simulink model "TVModel_Simulation"  (R2022a)
settings: Solver=FixedStepDiscrete  StartTime=0.0  StopTime=200  FixedStep=0.02  MaxStep=0.01  RelTol=1e-3
undefined symbols (not defined in the file or in its folder): TV
libraries: simulink x5, simulink_extras x3, dspstat3 x2, sharedTrackingLibrary x1, slpidlib x1, eeGeneralControl x1
(part 2 of 4)

== system TVModel_Simulation/Subsystem/Subsystem1/Slip Control/Slip Ratios/FR SR ==
  In Bus Element : Inport  PortName=dynamics_data  Element=omega_wheels
  In Bus Element4 : Inport  PortName=dynamics_data  Element=vx
  In Bus Element2 : Inport  PortName=dynamics_data  Element=vx
  In Bus Element1 : Inport  PortName=dynamics_data  Element=vy
  In Bus Element6 : Inport  Port=2  PortName=front_wheels_steering  Element=different_axis
  Constant : Constant  Value=0
  Cos1 : Trigonometry  Operator=cos
  Cos2 : Trigonometry
  Divide4 : Product  Inputs=*/
  Divide5 : Product  Inputs=**
  Divide6 : Product  Inputs=**
  Gain3 : Gain  Gain=TV.CAR.rs
  Selector : Selector  InputPortWidth=4  IndexOptions=Index vector (dialog)  Indices=[2]  OutputSizes=1
  Selector1 : Selector  InputPortWidth=2  IndexOptions=Index vector (dialog)  Indices=[2]  OutputSizes=1
  Subtract3 : Sum  Inputs=+-
  Sum : Sum
  Switch : Switch  Criteria=u2 > Threshold  Threshold=0.5  SaturateOnIntegerOverflow=off  InputSameDT=off
  FR : Outport
  wires:
  Constant/1 -> Switch/3
  Divide4/1 -> Switch/1  "FL"
  In Bus Element1/1 -> Divide6/2
  In Bus Element2/1 -> Divide5/1
  Divide6/1 -> Sum/2
  Gain3/1 -> Subtract3/1
  Divide5/1 -> Sum/1
  Cos1/1 -> Divide5/2
  Sum/1 -> Subtract3/2, Divide4/2
  Cos2/1 -> Divide6/1
  Subtract3/1 -> Divide4/1
  Switch/1 -> FR/1
  In Bus Element/1 -> Selector/1  "fr"
  Selector/1 -> Gain3/1
  In Bus Element4/1 -> Switch/2
  Selector1/1 -> Cos2/1, Cos1/1
  In Bus Element6/1 -> Selector1/1

== system TVModel_Simulation/Subsystem/Subsystem1/Slip Control/Slip Ratios/RL RR  ==
  In Bus Element : Inport  PortName=dynamics_data  Element=omega_wheels
  In Bus Element1 : Inport  PortName=dynamics_data  Element=vx
  Constant : Constant  Value=0
  Divide : Product  Inputs=*/
  Gain : Gain  Gain=TV.CAR.rs
  Selector : Selector  InputPortWidth=4  IndexOptions=Index vector (dialog)  Indices=[4]  OutputSizes=1
  Subtract : Sum  Inputs=+-
  Switch : Switch  Criteria=u2 > Threshold  Threshold=0.5  SaturateOnIntegerOverflow=off  InputSameDT=off
  RR : Outport
  wires:
  Constant/1 -> Switch/3
  Divide/1 -> Switch/1  "RL"
  Switch/1 -> RR/1  "RR"
  Gain/1 -> Subtract/1
  Subtract/1 -> Divide/1
  In Bus Element1/1 -> Switch/2, Divide/2, Subtract/2
  In Bus Element/1 -> Selector/1  "rr"
  Selector/1 -> Gain/1

== system TVModel_Simulation/Subsystem/Subsystem1/Slip Control/Slip Ratios/RL SR ==
  In Bus Element : Inport  PortName=dynamics_data  Element=omega_wheels
  In Bus Element1 : Inport  PortName=dynamics_data  Element=vx
  Constant : Constant  Value=0
  Divide : Product  Inputs=*/
  Gain : Gain  Gain=TV.CAR.rs
  Selector : Selector  InputPortWidth=4  IndexOptions=Index vector (dialog)  Indices=[3]  OutputSizes=1
  Subtract : Sum  Inputs=+-
  Switch : Switch  Criteria=u2 > Threshold  Threshold=0.5  SaturateOnIntegerOverflow=off  InputSameDT=off
  RL : Outport
  wires:
  In Bus Element1/1 -> Subtract/2, Divide/2, Switch/2
  Subtract/1 -> Divide/1
  Gain/1 -> Subtract/1
  Switch/1 -> RL/1  "RL"
  Divide/1 -> Switch/1  "RL"
  Constant/1 -> Switch/3
  In Bus Element/1 -> Selector/1  "rl"
  Selector/1 -> Gain/1

== system TVModel_Simulation/Subsystem/Subsystem1/Torque Distribution/MPC/     Output vector reference ==
  YRD : Inport
  In Bus Element1 : Inport  Port=2  PortName=dynamics_data  Element=vy
  In Bus Element : Inport  Port=2  PortName=dynamics_data  Element=vx
  In Bus Element3 : Inport  Port=2  PortName=dynamics_data  Element=vx
  In Bus Element2 : Inport  Port=3  PortName=driver_inputs  Element=throttle
  Bus Creator : BusCreator  Inputs=11
  Bus y_ref : Subsystem
  MATLAB Function : MATLAB Function  TreatAsAtomicUnit=on
  MATLAB Function1 : MATLAB Function  TreatAsAtomicUnit=on
  T_FL_ref : Constant  Value=0
  T_FR_ref : Constant  Value=0
  T_RL_ref : Constant  Value=0
  T_RR_ref : Constant  Value=0
  YRD1 : InportShadow
  dT_FL_ref : Constant  Value=0
  dT_FR_ref : Constant  Value=0
  dT_RL_ref : Constant  Value=0
  dT_RR_ref : Constant  Value=0
  y_ref_0 : Outport
  y_ref : Outport  Port=2
  Out Bus Element5 : Outport  Port=3  PortName=TV_Info  Element=vx_ref
  Out Bus Element1 : Outport  Port=3  PortName=TV_Info  Element=vy_ref
  wires:
  dT_RR_ref/1 -> Bus Creator/11
  dT_RL_ref/1 -> Bus Creator/10
  dT_FR_ref/1 -> Bus Creator/9
  dT_FL_ref/1 -> Bus Creator/8
  In Bus Element2/1 -> MATLAB Function1/3(acc)
  In Bus Element1/1 -> MATLAB Function1/2(vy)
  In Bus Element/1 -> MATLAB Function1/1(vx)
  MATLAB Function1/1(vx_ref) -> Bus Creator/1, Out Bus Element5/1  "vx_ref"
  MATLAB Function/1(vy_ref) -> Bus Creator/2, Out Bus Element1/1  "vy_ref"
  T_FL_ref/1 -> Bus Creator/4
  T_FR_ref/1 -> Bus Creator/5
  T_RL_ref/1 -> Bus Creator/6
  T_RR_ref/1 -> Bus Creator/7
  Bus Creator/1 -> Bus y_ref/1(u), y_ref_0/1
  Bus y_ref/1(y) -> y_ref/1
  In Bus Element3/1 -> MATLAB Function/1(vx)
  YRD/1 -> MATLAB Function/2(YRD)  "r_ref"
  YRD1/1 -> Bus Creator/3  "r_ref"

== system TVModel_Simulation/Subsystem/Subsystem1/Torque Distribution/MPC/ Parameter Bus  ==
  note: Nominal LMU = 0.93
  In Bus Element1 : Inport  PortName=slip_ratio  Element=fl
  In Bus Element2 : Inport  PortName=slip_ratio  Element=fr
  In Bus Element3 : Inport  PortName=slip_ratio  Element=rl
  In Bus Element4 : Inport  PortName=slip_ratio  Element=rr
  In Bus Element5 : Inport  Port=2  PortName=dynamics_data  Element=ax
  In Bus Element6 : Inport  Port=2  PortName=dynamics_data  Element=ay
  In Bus Element12 : Inport  Port=2  PortName=dynamics_data  Element=brake_torque
  In Bus Element11 : Inport  Port=3  PortName=front_wheel_angles  Element=single_axis
  Bus p : Subsystem
  Demux : Demux
  Inertia Scaling : Constant
  LMUy : Constant  Value=0.93
  Mux : Mux  Inputs=TV.MPC.np
  Signal Specification{4..7} (4 alike) : SignalSpecification  Dimensions=1
  p : Outport
  wires:
  Inertia Scaling/1 -> Mux/13
  In Bus Element11/1 -> Mux/1
  LMUy/1 -> Mux/12
  Bus p/1(Out) -> p/1
  Demux/1 -> Signal Specification4/1
  Demux/2 -> Signal Specification5/1
  Demux/3 -> Signal Specification6/1
  Demux/4 -> Signal Specification7/1
  Signal Specification4/1 -> Mux/6
  Signal Specification5/1 -> Mux/7
  Signal Specification6/1 -> Mux/8
  Signal Specification7/1 -> Mux/9
  Mux/1 -> Bus p/1(In)
  In Bus Element1/1 -> Mux/2
  In Bus Element4/1 -> Mux/5
  In Bus Element3/1 -> Mux/4
  In Bus Element2/1 -> Mux/3
  In Bus Element6/1 -> Mux/10
  In Bus Element5/1 -> Mux/11
  In Bus Element12/1 -> Demux/1

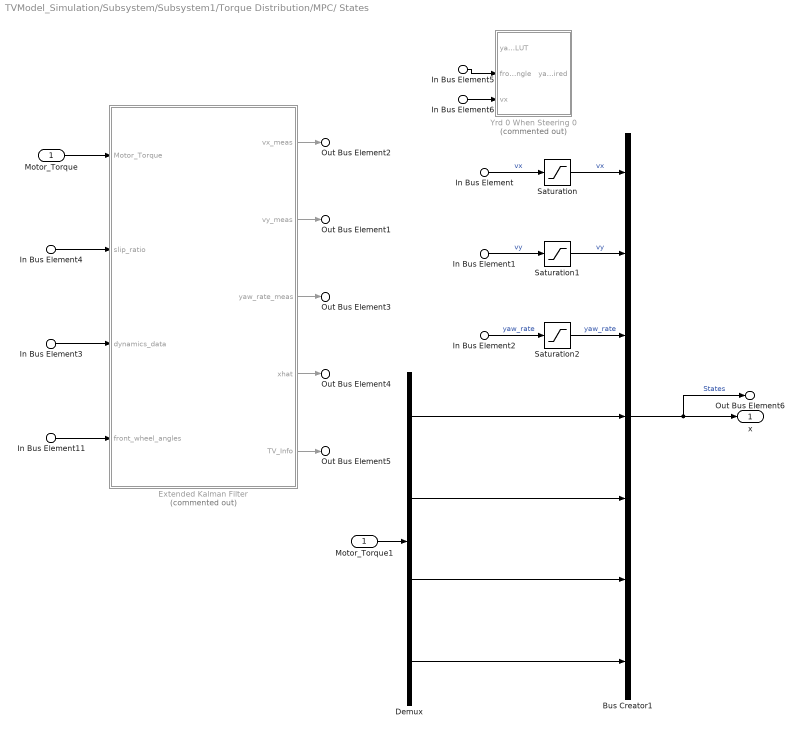
== system TVModel_Simulation/Subsystem/Subsystem1/Torque Distribution/MPC/ States ==
  Motor_Torque : Inport
  In Bus Element4 : Inport  Port=2  PortName=slip_ratio
  In Bus Element3 : Inport  Port=3  PortName=dynamics_data
  In Bus Element : Inport  Port=3  PortName=dynamics_data  Element=vx
  In Bus Element6 : Inport  Port=3  PortName=dynamics_data  Element=vx
  In Bus Element1 : Inport  Port=3  PortName=dynamics_data  Element=vy
  In Bus Element2 : Inport  Port=3  PortName=dynamics_data  Element=yaw_rate
  In Bus Element11 : Inport  Port=4  PortName=front_wheel_angles
  In Bus Element5 : Inport  Port=4  PortName=front_wheel_angles  Element=single_axis
  Bus Creator1 : BusCreator  Inputs=7
  Demux : Demux
  Extended Kalman Filter : Subsystem  Commented=on
  Motor_Torque1 : InportShadow
  Saturation : Saturate  UpperLimit=inf  LowerLimit=2
  Saturation1 : Saturate  UpperLimit=5  LowerLimit=-5
  Saturation2 : Saturate  UpperLimit=4  LowerLimit=-4
  Yrd 0 When Steering 0 : Subsystem  Commented=on
      mask Display: image('Mask_Icon\On_Off.png'); % Use "Edit Image" on toolstrip to change.
  x : Outport
  Out Bus Element4 : Outport  Port=2  PortName=TV_Info  Element=xhat
  Out Bus Element5 : Outport  Port=2  PortName=TV_Info  Element=EKF
  Out Bus Element3 : Outport  Port=2  PortName=TV_Info  Element=r_meas
  Out Bus Element1 : Outport  Port=2  PortName=TV_Info  Element=vy_meas
  Out Bus Element2 : Outport  Port=2  PortName=TV_Info  Element=vx_meas
  Out Bus Element6 : Outport  Port=2  PortName=TV_Info  Element=x
  wires:
  Demux/4 -> Bus Creator1/7
  Demux/3 -> Bus Creator1/6
  Demux/2 -> Bus Creator1/5
  Demux/1 -> Bus Creator1/4
  Motor_Torque1/1 -> Demux/1
  In Bus Element5/1 -> Yrd 0 When Steering 0/2(front_steer_angle)
  In Bus Element11/1 -> Extended Kalman Filter/4(front_wheel_angles)
  Motor_Torque/1 -> Extended Kalman Filter/1(Motor_Torque)
  In Bus Element4/1 -> Extended Kalman Filter/2(slip_ratio)
  In Bus Element3/1 -> Extended Kalman Filter/3(dynamics_data)
  Extended Kalman Filter/3(yaw_rate_meas) -> Out Bus Element3/1
  Extended Kalman Filter/1(vx_meas) -> Out Bus Element2/1
  Extended Kalman Filter/2(vy_meas) -> Out Bus Element1/1
  In Bus Element2/1 -> Saturation2/1  "yaw_rate"
  Saturation/1 -> Bus Creator1/1  "vx"
  In Bus Element1/1 -> Saturation1/1  "vy"
  In Bus Element/1 -> Saturation/1  "vx"
  Extended Kalman Filter/4(xhat) -> Out Bus Element4/1
  Bus Creator1/1 -> x/1, Out Bus Element6/1  "States"
  Extended Kalman Filter/5(TV_Info) -> Out Bus Element5/1
  In Bus Element6/1 -> Yrd 0 When Steering 0/3(vx)
  Saturation1/1 -> Bus Creator1/2  "vy"
  Saturation2/1 -> Bus Creator1/3  "yaw_rate"

== system TVModel_Simulation/Subsystem/Subsystem1/Torque Distribution/MPC/Control Constraints ==
  Constant : Constant  Value=1000*ones(4,1)
  Unary Minus : UnaryMinus
  lbu : Outport
  ubu : Outport  Port=2
  wires:
  Unary Minus/1 -> lbu/1
  Constant/1 -> ubu/1, Unary Minus/1

== system TVModel_Simulation/Subsystem/Subsystem1/Torque Distribution/MPC/ESP ==
  In Bus Element : Inport  PortName=driver_inputs  Element=throttle
  In Bus Element32 : Inport  Port=2  PortName=brake_signal  Element=regen
  AND : Logic  IconShape=distinctive  AllPortsSameDT=off  OutDataTypeStr=boolean
  Constant1 : Constant  Value=TV.LV.GENERAL.BrakeThresh
  Constant2 : Constant  Value=TV.LV.GENERAL.ThrottleThresh
  Less Than : RelationalOperator  Operator=<  OutDataTypeStr=boolean  RndMeth=Simplest  InputSameDT=off
  Less Than1 : RelationalOperator  Operator=>  OutDataTypeStr=boolean  RndMeth=Simplest  InputSameDT=off
  ESP_Flag : Outport
  wires:
  In Bus Element/1 -> Less Than/1
  In Bus Element32/1 -> Less Than1/2
  Less Than/1 -> AND/1
  Less Than1/1 -> AND/2
  AND/1 -> ESP_Flag/1
  Constant1/1 -> Less Than1/1
  Constant2/1 -> Less Than/2

== system TVModel_Simulation/Subsystem/Subsystem1/Torque Distribution/MPC/Faults detection ==
  Control : Inport
  OCP Status : Inport  Port=2
  In Bus Element : Inport  Port=3  PortName=dynamics_data
  In Bus Element5 : Inport  Port=3  PortName=dynamics_data
  In Bus Element3 : Inport  Port=3  PortName=dynamics_data  Element=omega_wheels
  In Bus Element1 : Inport  Port=4  PortName=driver_inputs
  In Bus Element2 : Inport  Port=4  PortName=driver_inputs  Element=brake
  Power flag : Subsystem  Commented=on
  Subsystem : Subsystem  Commented=on
  Subsystem2 : Subsystem
  Switch : Switch  Criteria=u2 > Threshold  SaturateOnIntegerOverflow=off  InputSameDT=off
  Switch2 : Switch  Commented=on  Criteria=u2 > Threshold  SaturateOnIntegerOverflow=off  InputSameDT=off
  Motor_Torque : Outport
  wires:
  Power flag/1(Output) -> Switch2/2
  Subsystem/1(Output) -> Switch2/1
  In Bus Element5/1 -> Power flag/2(dynamics_data)
  In Bus Element2/1 -> Subsystem/3(In3)
  In Bus Element3/1 -> Subsystem/2(In2)
  Subsystem2/2(flag) -> Switch/2  "flag"
  Subsystem2/1(Simple Torque) -> Switch/1
  Switch/1 -> Subsystem/1(T), Power flag/1(Motor_Torque), Motor_Torque/1
  Control/1 -> Switch/3
  In Bus Element1/1 -> Subsystem2/2(driver_inputs)
  In Bus Element/1 -> Subsystem2/1(dynamics_data)  "vx"
  OCP Status/1 -> Subsystem2/3(OCP Status)

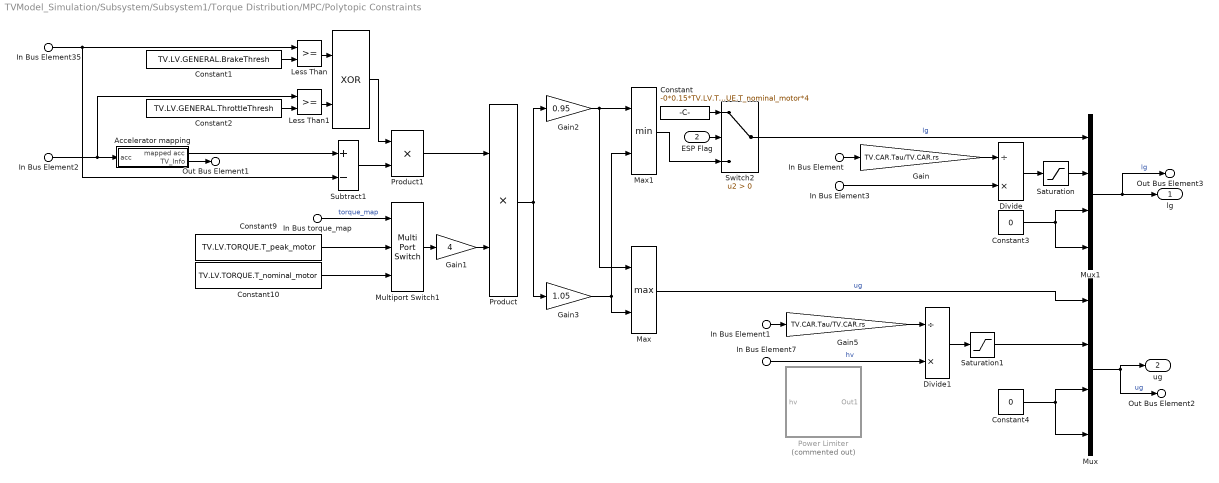
== system TVModel_Simulation/Subsystem/Subsystem1/Torque Distribution/MPC/Polytopic Constraints ==
  In Bus Element : Inport  PortName=dynamics_data  Element=vx
  In Bus Element1 : Inport  PortName=dynamics_data  Element=vx
  ESP Flag : Inport  Port=2
  In Bus Element35 : Inport  Port=3  PortName=brake_signal  Element=regen
  In Bus Element2 : Inport  Port=4  PortName=driver_inputs  Element=throttle
  In Bus torque_map : Inport  Port=5  PortName=Car_Settings  Element=torque_map
  In Bus Element3 : Inport  Port=6  PortName=hv  Element=Pmax_regen
  In Bus Element7 : Inport  Port=6  PortName=hv  Element=Pmax_tractive
  " " : Logic  Operator=XOR  IconShape=distinctive  AllPortsSameDT=off  OutDataTypeStr=boolean
  "Accelerator mapping " : Subsystem
  Constant : Constant  Value=-0*0.15*TV.LV.TORQUE.T_nominal_motor*4
  Constant1 : Constant  Value=TV.LV.GENERAL.BrakeThresh
  Constant10 : Constant  Value=TV.LV.TORQUE.T_nominal_motor
  Constant2 : Constant  Value=TV.LV.GENERAL.ThrottleThresh
  Constant3 : Constant  Value=0
  Constant4 : Constant  Value=0
  Constant9 : Constant  Value=TV.LV.TORQUE.T_peak_motor
  Divide : Product  Inputs=/*
  Divide1 : Product  Inputs=/*
  Gain : Gain  Gain=TV.CAR.Tau/TV.CAR.rs
  Gain1 : Gain  Gain=4
  Gain2 : Gain  Gain=0.95
  Gain3 : Gain  Gain=1.05
  Gain5 : Gain  Gain=TV.CAR.Tau/TV.CAR.rs
  Less Than : RelationalOperator  OutDataTypeStr=boolean  RndMeth=Simplest  InputSameDT=off
  Less Than1 : RelationalOperator  OutDataTypeStr=boolean  RndMeth=Simplest  InputSameDT=off
  Max : MinMax  Function=max  Inputs=2
  Max1 : MinMax  Inputs=2
  Multiport Switch1 : MultiPortSwitch  DataPortOrder=Specify indices  Inputs={TV.LV.TORQUE.T_peak_setting,TV.LV.TORQUE.T_nominal_setting}  DataPortIndices={TV.LV.TORQUE.T_peak_setting,TV.LV.TORQUE.T_nominal_setting}  SaturateOnIntegerOverflow=off  InputSameDT=off
  Mux : Mux
  Mux1 : Mux
  Power Limiter : Subsystem  Commented=on
  Product : Product
  Product1 : Product
  Saturation : Saturate  UpperLimit=0  LowerLimit=-10*TV.LV.TORQUE.T_peak_motor
  Saturation1 : Saturate  UpperLimit=10*TV.LV.TORQUE.T_peak_motor  LowerLimit=0
  Subtract1 : Sum  Inputs=+-
  Switch2 : Switch  Criteria=u2 > Threshold  SaturateOnIntegerOverflow=off  InputSameDT=off
  lg : Outport
  ug : Outport  Port=2
  Out Bus Element1 : Outport  Port=3  PortName=TV_Info  Element=Accelerator_Mapping
  Out Bus Element2 : Outport  Port=3  PortName=TV_Info  Element=ug
  Out Bus Element3 : Outport  Port=3  PortName=TV_Info  Element=lg
  wires:
  Saturation/1 -> Mux1/2
  Saturation1/1 -> Mux/2
  Product1/1 -> Product/1
  Multiport Switch1/1 -> Gain1/1
  In Bus torque_map/1 -> Multiport Switch1/1  "torque_map"
  Constant10/1 -> Multiport Switch1/3
  Constant9/1 -> Multiport Switch1/2
  Gain/1 -> Divide/1
  In Bus Element3/1 -> Divide/2
  Divide1/1 -> Saturation1/1
  Divide/1 -> Saturation/1
  Switch2/1 -> Mux1/1  "lg"
  Constant2/1 -> Less Than1/2
  Constant1/1 -> Less Than/2
  In Bus Element35/1 -> Less Than/1, Subtract1/2
  In Bus Element2/1 -> "Accelerator mapping "/1(acc), Less Than1/1
  "Accelerator mapping "/1(mapped acc) -> Subtract1/1
  " "/1 -> Product1/1
  Less Than1/1 -> " "/2
  Less Than/1 -> " "/1
  Subtract1/1 -> Product1/2
  In Bus Element1/1 -> Gain5/1
  Gain5/1 -> Divide1/1
  Max/1 -> Mux/1  "ug"
  Mux/1 -> Out Bus Element2/1, ug/1  "ug"
  Mux1/1 -> Out Bus Element3/1, lg/1  "lg"
  In Bus Element/1 -> Gain/1
  Constant/1 -> Switch2/1
  ESP Flag/1 -> Switch2/2
  Constant3/1 -> Mux1/3, Mux1/4
  Constant4/1 -> Mux/3, Mux/4
  "Accelerator mapping "/2(TV_Info) -> Out Bus Element1/1
  Gain1/1 -> Product/2
  Product/1 -> Gain2/1, Gain3/1
  Max1/1 -> Switch2/3
  Gain3/1 -> Max/2, Max1/2
  Gain2/1 -> Max/1, Max1/1
  In Bus Element7/1 -> Divide1/2  "hv"

== system TVModel_Simulation/Subsystem/Subsystem1/Torque Distribution/MPC/Polytropic Matrix ==
  In Bus Element1 : Inport  PortName=dynamics_data
  Torque : Inport  Port=2
  Efficiency limit : Subsystem
  MATLAB Function : MATLAB Function  TreatAsAtomicUnit=on
  C : Outport
  wires:
  MATLAB Function/1(y) -> C/1  "C"
  Efficiency limit/1(Limit) -> MATLAB Function/1(Limit)  "Limit"
  In Bus Element1/1 -> Efficiency limit/2(dynamics_data)
  Torque/1 -> Efficiency limit/1(Motor_Torque)

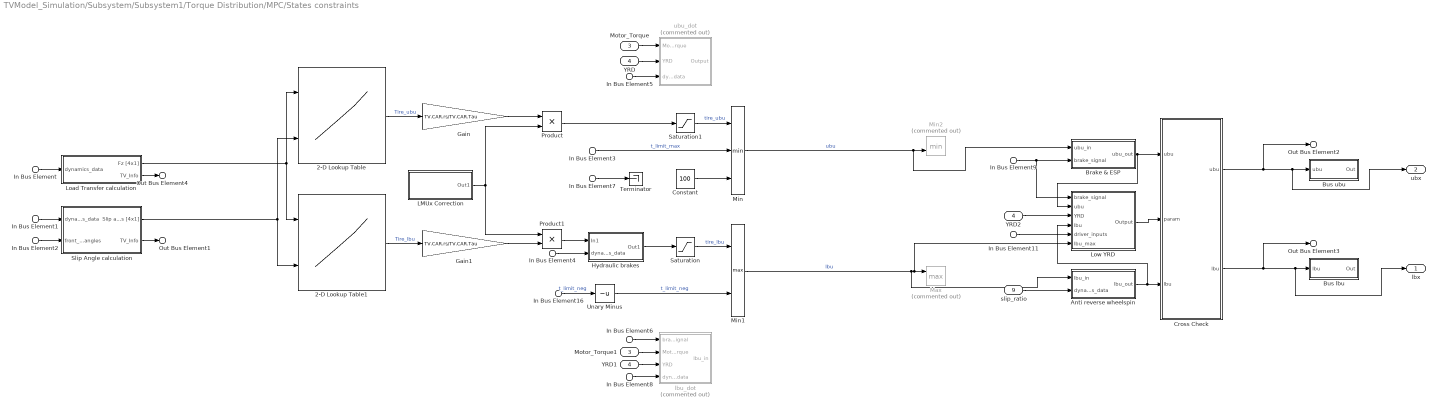
== system TVModel_Simulation/Subsystem/Subsystem1/Torque Distribution/MPC/States constraints ==
  In Bus Element2 : Inport  PortName=front_wheel_angles
  In Bus Element16 : Inport  Port=2  PortName=mpc_torque_limit  Element=t_limit_negative
  In Bus Element3 : Inport  Port=2  PortName=mpc_torque_limit  Element=t_limit_positive
  Motor_Torque : Inport  Port=3
  YRD : Inport  Port=4
  In Bus Element9 : Inport  Port=5  PortName=brake_signal
  In Bus Element6 : Inport  Port=5  PortName=brake_signal
  In Bus Element7 : Inport  Port=6  PortName=TC_Torque
  In Bus Element{,1,4..5,8} (5 alike) : Inport  Port=7  PortName=dynamics_data
  In Bus Element11 : Inport  Port=8  PortName=driver_inputs
  slip_ratio : Inport  Port=9
  2-D Lookup Table : Lookup_n-D  BreakpointsForDimension1=TV.LUT.MPC_Lut.control_bound_0_10.Fz  BreakpointsForDimension2=TV.LUT.MPC_Lut.control_bound_0_10.alpha  Table=TV.LUT.MPC_Lut.control_bound_0_10.Fx_target_positive  InternalRulePriority=Speed  RndMeth=Simplest
      settings: InputPortMap=u0,u1
  2-D Lookup Table1 : Lookup_n-D  BreakpointsForDimension1=TV.LUT.MPC_Lut.control_bound_0_10.Fz  BreakpointsForDimension2=TV.LUT.MPC_Lut.control_bound_0_10.alpha  Table=TV.LUT.MPC_Lut.control_bound_0_10.Fx_target_negative  InternalRulePriority=Speed  RndMeth=Simplest
      settings: InputPortMap=u0,u1
  Anti reverse wheelspin : Subsystem
  Brake & ESP : Subsystem
  Bus lbu : Subsystem
  Bus ubu : Subsystem
  Constant : Constant  Value=100
  Cross Check : MATLAB Function  TreatAsAtomicUnit=on
  Gain : Gain  Gain=TV.CAR.rs/TV.CAR.Tau
  Gain1 : Gain  Gain=TV.CAR.rs/TV.CAR.Tau
  Hydraulic brakes : Subsystem
  LMUx Correction : Subsystem
  Load Transfer calculation : Subsystem
  Low YRD : Subsystem
  Max : MinMax  Commented=on  Function=max  Inputs=2
  Min : MinMax  Inputs=3
  Min1 : MinMax  Function=max  Inputs=2
  Min2 : MinMax  Commented=on  Inputs=2
  Motor_Torque1 : InportShadow  Port=3
  Product : Product
  Product1 : Product
  Saturation : Saturate  UpperLimit=0  LowerLimit=-inf
  Saturation1 : Saturate  UpperLimit=+inf  LowerLimit=0
  Slip Angle calculation : Subsystem
  Terminator : Terminator
  Unary Minus : UnaryMinus
  YRD1 : InportShadow  Port=4
  YRD2 : InportShadow  Port=4
  lbu_dot : Subsystem  Commented=on
  ubu_dot : Subsystem  Commented=on
  lbx : Outport
  ubx : Outport  Port=2
  Out Bus Element4 : Outport  Port=3  PortName=TV_Info  Element=Load_Transfer_Calculation
  Out Bus Element1 : Outport  Port=3  PortName=TV_Info  Element=Slip_Angle_Calculation
  Out Bus Element2 : Outport  Port=3  PortName=TV_Info  Element=ubu
  Out Bus Element3 : Outport  Port=3  PortName=TV_Info  Element=lbu
  wires:
  YRD/1 -> ubu_dot/2(YRD)
  Min1/1 -> Low YRD/6(lbu_max), Max/1, Anti reverse wheelspin/1(lbu_in)  "lbu"
  In Bus Element11/1 -> Low YRD/5(driver_inputs)
  YRD2/1 -> Low YRD/3(YRD)
  slip_ratio/1 -> Anti reverse wheelspin/2(dynamics_data)
  In Bus Element9/1 -> Brake & ESP/2(brake_signal), Low YRD/1(brake_signal)
  In Bus Element8/1 -> lbu_dot/4(dynamics_data)
  YRD1/1 -> lbu_dot/3(YRD)
  Motor_Torque1/1 -> lbu_dot/2(Motor_Torque)
  In Bus Element6/1 -> lbu_dot/1(brake_signal)
  In Bus Element5/1 -> ubu_dot/3(dynamics_data)
  Motor_Torque/1 -> ubu_dot/1(Motor_Torque)
  In Bus Element4/1 -> Hydraulic brakes/2(dynamics_data)
  In Bus Element2/1 -> Slip Angle calculation/2(front_wheel_angles)
  In Bus Element1/1 -> Slip Angle calculation/1(dynamics_data)
  In Bus Element/1 -> Load Transfer calculation/1(dynamics_data)
  Low YRD/1(Output) -> Cross Check/2(param)
  Min/1 -> Min2/2, Brake & ESP/1(ubu_in)  "ubu"
  Anti reverse wheelspin/1(lbu_out) -> Low YRD/4(lbu), Cross Check/3("lbu ")
  Brake & ESP/1(ubu_out) -> Low YRD/2(ubu), Cross Check/1("ubu ")
  LMUx Correction/1(Out1) -> Product1/1, Product/2
  Product1/1 -> Hydraulic brakes/1(In1)
  Gain1/1 -> Product1/2
  Gain/1 -> Product/1
  Hydraulic brakes/1(Out1) -> Saturation/1
  Load Transfer calculation/1(Fz [4x1]) -> 2-D Lookup Table1/1, 2-D Lookup Table/1
  2-D Lookup Table/1 -> Gain/1  "Tire_ubu"
  2-D Lookup Table1/1 -> Gain1/1  "Tire_lbu"
  Slip Angle calculation/1(Slip angles [4x1]) -> 2-D Lookup Table1/2, 2-D Lookup Table/2
  In Bus Element3/1 -> Min/2  "t_limit_max"
  In Bus Element16/1 -> Unary Minus/1  "t_limit_neg"
  Load Transfer calculation/2(TV_Info) -> Out Bus Element4/1
  Slip Angle calculation/2(TV_Info) -> Out Bus Element1/1
  Product/1 -> Saturation1/1
  Cross Check/1(ubu) -> Out Bus Element2/1, Bus ubu/1(ubu), ubx/1
  Cross Check/2(lbu) -> Out Bus Element3/1, Bus lbu/1(lbu), lbx/1
  Unary Minus/1 -> Min1/2  "t_limit_neg"
  Saturation/1 -> Min1/1  "tire_lbu"
  Saturation1/1 -> Min/1  "tire_ubu"
  In Bus Element7/1 -> Terminator/1
  Constant/1 -> Min/3

== system TVModel_Simulation/Subsystem/Subsystem1/Torque Distribution/MPC/Subsystem ==
  In1 : Inport
  Demux : Demux  Outputs=7
  Mux : Mux
  Selector : Selector  Commented=on  InputPortWidth=7  IndexOptions=Index vector (dialog)  Indices=[4:7]  OutputSizes=1
  Terminator : Terminator
  Terminator1 : Terminator
  Terminator2 : Terminator
  Control : Outport
  wires:
  Mux/1 -> Control/1
  Demux/3 -> Terminator2/1
  Demux/2 -> Terminator1/1
  Demux/1 -> Terminator/1
  Demux/5 -> Mux/2
  Demux/6 -> Mux/3
  Demux/7 -> Mux/4
  Demux/4 -> Mux/1
  In1/1 -> Selector/1, Demux/1

== system TVModel_Simulation/Subsystem/Subsystem1/Torque Distribution/MPC/Weights generation ==
  In Bus Element30 : Inport  PortName=front_wheel_angles  Element=single_axis
  Torque : Inport  Port=2
  In Bus Element1 : Inport  Port=3  PortName=dynamics_data
  Constant : Constant  Value=1*ones(4,1)
  Constant1 : Constant  Commented=on  Value=1e-2*ones(4,1)
  Demux : Demux
  Demux1 : Demux
  Efficiency limit : Subsystem
  Gain : Gain  Gain=1e-2
  MATLAB Function : MATLAB Function  TreatAsAtomicUnit=on
  Mux : Mux  Inputs=TV.MPC.ny
  Non-Linear Activation : MATLAB Function  TreatAsAtomicUnit=on
  Subsystem1 : Subsystem  Commented=on
  r1 : Constant  Value=100
  r2 : Constant  Value=0
  vx : Constant  Value=0
  vy : Constant  Value=10
  y : Outport
  wires:
  Efficiency limit/1(Limit) -> Gain/1  "Limit"
  Demux1/2 -> Mux/9
  Demux1/4 -> Mux/11
  Demux1/1 -> Mux/8
  Constant/1 -> Demux1/1
  Demux1/3 -> Mux/10
  Mux/1 -> MATLAB Function/1(u)
  vy/1 -> Mux/2
  vx/1 -> Mux/1
  MATLAB Function/1(y) -> y/1
  r2/1 -> Non-Linear Activation/3(in_2)
  r1/1 -> Non-Linear Activation/1(in_1), Mux/3
  In Bus Element30/1 -> Subsystem1/1(front_wheel_angles)
  Subsystem1/1(epsilon) -> Non-Linear Activation/2(epsilon)
  Demux/1 -> Mux/4
  Demux/2 -> Mux/5
  Demux/4 -> Mux/7
  Demux/3 -> Mux/6
  Torque/1 -> Efficiency limit/1(Motor_Torque)
  In Bus Element1/1 -> Efficiency limit/2(dynamics_data)
  Gain/1 -> Demux/1

== system TVModel_Simulation/Subsystem/Subsystem1/Torque Distribution/Reference Tracking/Subsystem ==
  In1 : Inport
  Abs : Abs  SaturateOnIntegerOverflow=off
  Constant : Constant  Value=1*pi/180
  Gain : Gain  Gain=1/(2*pi/180)
  Saturation : Saturate  UpperLimit=1  LowerLimit=0
  Saturation1 : Saturate  UpperLimit=inf  LowerLimit=0
  Subtract : Sum  Inputs=+-
  epsilon : Outport
  wires:
  Subtract/1 -> Saturation1/1
  Gain/1 -> Saturation/1
  Saturation/1 -> epsilon/1
  In1/1 -> Abs/1
  Constant/1 -> Subtract/2
  Saturation1/1 -> Gain/1
  Abs/1 -> Subtract/1

== system TVModel_Simulation/Subsystem/Subsystem1/Torque Distribution/Reference Tracking/YRD_LUT_-1 ==
  front_wheel_angle : Inport
  vx : Inport  Port=2
  Action Port : ActionPort  ActionPortLabel=elseif(u1 ==4)
  Abs : Abs  SaturateOnIntegerOverflow=off
  Cast3 : DataTypeConversion  Commented=on  OutDataTypeStr=single  SaturateOnIntegerOverflow=off  RndMeth=Floor
  Divide : Product  Inputs=*/
  Divide1 : Product  Inputs=*/
  Divide2 : Product  Inputs=**
  LUT_-3 : Lookup_n-D  BreakpointsForDimension1=TV.LUT.Yrd_LUT.LUT_vectors.delta_vector  BreakpointsForDimension2=TV.LUT.Yrd_LUT.LUT_vectors.v_vector  Table=single(TV.LUT.Yrd_LUT.LUT_neg3.ay_matrix)  InternalRulePriority=Speed  RndMeth=Simplest
      settings: InputPortMap=u0,u1
  Saturation : Saturate  UpperLimit=inf  LowerLimit=3
  yrd : Outport
  wires:
  front_wheel_angle/1 -> Divide1/1, Abs/1
  Abs/1 -> Divide1/2, LUT_-3/1  "absolute_front_wheel_angle"
  Divide/1 -> Divide2/2
  LUT_-3/1 -> Divide/1  "a"
  vx/1 -> Saturation/1
  Saturation/1 -> Divide/2, LUT_-3/2  "vx"
  Divide2/1 -> yrd/1  "yrd"
  Divide1/1 -> Divide2/1  "normalized_front_wheel_angle"

== system TVModel_Simulation/Subsystem/Subsystem1/Torque Distribution/Reference Tracking/YRD_LUT_-1.1 ==
  front_wheel_angle : Inport
  vx : Inport  Port=2
  Action Port : ActionPort  ActionPortLabel=elseif(u1 ==3)
  Abs : Abs  SaturateOnIntegerOverflow=off
  Cast3 : DataTypeConversion  Commented=on  OutDataTypeStr=single  SaturateOnIntegerOverflow=off  RndMeth=Floor
  Divide : Product  Inputs=*/
  Divide1 : Product  Inputs=*/
  Divide2 : Product  Inputs=**
  LUT_-1.5 : Lookup_n-D  BreakpointsForDimension1=TV.LUT.Yrd_LUT.LUT_vectors.delta_vector  BreakpointsForDimension2=TV.LUT.Yrd_LUT.LUT_vectors.v_vector  Table=single(TV.LUT.Yrd_LUT.LUT_neg1_5.ay_matrix)  InternalRulePriority=Speed  RndMeth=Simplest
      settings: InputPortMap=u0,u1
  Saturation : Saturate  UpperLimit=inf  LowerLimit=3
  yrd : Outport
  wires:
  front_wheel_angle/1 -> Divide1/1, Abs/1
  vx/1 -> Saturation/1
  Divide1/1 -> Divide2/1  "normalized_front_wheel_angle"
  Divide2/1 -> yrd/1  "yrd"
  Abs/1 -> Divide1/2, LUT_-1.5/1  "absolute_front_wheel_angle"
  Saturation/1 -> Divide/2, LUT_-1.5/2  "vx"
  LUT_-1.5/1 -> Divide/1
  Divide/1 -> Divide2/2

== system TVModel_Simulation/Subsystem/Subsystem1/Torque Distribution/Reference Tracking/YRD_LUT_-1.5 ==
  front_wheel_angle : Inport
  vx : Inport  Port=2
  Action Port : ActionPort
  Abs : Abs  SaturateOnIntegerOverflow=off
  Cast3 : DataTypeConversion  Commented=on  OutDataTypeStr=single  SaturateOnIntegerOverflow=off  RndMeth=Floor
  Divide : Product  Inputs=*/
  Divide1 : Product  Inputs=*/
  Divide2 : Product  Inputs=**
  LUT_-1.5 : Lookup_n-D  BreakpointsForDimension1=TV.LUT.Yrd_LUT.LUT_vectors.delta_vector  BreakpointsForDimension2=TV.LUT.Yrd_LUT.LUT_vectors.v_vector  Table=single(TV.LUT.Yrd_LUT.LUT_neg1_5.ay_matrix)  InternalRulePriority=Speed  RndMeth=Simplest
      settings: InputPortMap=u0,u1
  Saturation : Saturate  UpperLimit=inf  LowerLimit=3
  yrd : Outport
  wires:
  Divide/1 -> Divide2/2
  LUT_-1.5/1 -> Divide/1
  Saturation/1 -> LUT_-1.5/2, Divide/2  "vx"
  Abs/1 -> LUT_-1.5/1, Divide1/2  "absolute_front_wheel_angle"
  Divide2/1 -> yrd/1  "yrd"
  Divide1/1 -> Divide2/1  "normalized_front_wheel_angle"
  vx/1 -> Saturation/1
  front_wheel_angle/1 -> Abs/1, Divide1/1

== system TVModel_Simulation/Subsystem/Subsystem1/Torque Distribution/Reference Tracking/YRD_LUT_-3 ==
  front_wheel_angle : Inport
  vx : Inport  Port=2
  Action Port : ActionPort
  Abs : Abs  SaturateOnIntegerOverflow=off
  Cast3 : DataTypeConversion  Commented=on  OutDataTypeStr=single  SaturateOnIntegerOverflow=off  RndMeth=Floor
  Divide : Product  Inputs=*/
  Divide1 : Product  Inputs=*/
  Divide2 : Product  Inputs=**
  LUT_-3 : Lookup_n-D  BreakpointsForDimension1=TV.LUT.Yrd_LUT.LUT_vectors.delta_vector  BreakpointsForDimension2=TV.LUT.Yrd_LUT.LUT_vectors.v_vector  Table=single(TV.LUT.Yrd_LUT.LUT_neg3.ay_matrix)  InternalRulePriority=Speed  RndMeth=Simplest
      settings: InputPortMap=u0,u1
  Saturation : Saturate  UpperLimit=inf  LowerLimit=3
  yrd : Outport
  wires:
  Divide1/1 -> Divide2/1  "normalized_front_wheel_angle"
  Divide2/1 -> yrd/1  "yrd"
  Saturation/1 -> LUT_-3/2, Divide/2  "vx"
  vx/1 -> Saturation/1
  LUT_-3/1 -> Divide/1  "a"
  Divide/1 -> Divide2/2
  Abs/1 -> LUT_-3/1, Divide1/2  "absolute_front_wheel_angle"
  front_wheel_angle/1 -> Abs/1, Divide1/1

== system TVModel_Simulation/Subsystem/Subsystem1/Torque Distribution/Reference Tracking/YRD_LUT_0 ==
  front_wheel_angle : Inport
  vx : Inport  Port=2
  Action Port : ActionPort
  Abs : Abs  SaturateOnIntegerOverflow=off
  Cast : DataTypeConversion  Commented=on  OutDataTypeStr=single  SaturateOnIntegerOverflow=off  RndMeth=Floor
  Divide : Product  Inputs=*/
  Divide1 : Product  Inputs=*/
  Divide2 : Product  Inputs=**
  LUT_0 : Lookup_n-D  BreakpointsForDimension1=TV.LUT.Yrd_LUT.LUT_vectors.delta_vector  BreakpointsForDimension2=TV.LUT.Yrd_LUT.LUT_vectors.v_vector  Table=single(TV.LUT.Yrd_LUT.LUT_0.ay_matrix)  InternalRulePriority=Speed  RndMeth=Simplest
      settings: InputPortMap=u0,u1
  Saturation : Saturate  UpperLimit=inf  LowerLimit=3
  yrd : Outport
  wires:
  LUT_0/1 -> Divide/1
  Divide1/1 -> Divide2/1  "normalized_front_wheel_angle"
  Divide/1 -> Divide2/2
  vx/1 -> Saturation/1
  Divide2/1 -> yrd/1  "yrd"
  Abs/1 -> LUT_0/1, Divide1/2  "absolute_front_wheel_angle"
  Saturation/1 -> LUT_0/2, Divide/2  "vx"
  front_wheel_angle/1 -> Abs/1, Divide1/1

== system TVModel_Simulation/Subsystem/Subsystem1/Torque Distribution/Reference Tracking/YRD_LUT_1 ==
  front_wheel_angle : Inport
  vx : Inport  Port=2
  Action Port : ActionPort
  Abs : Abs  SaturateOnIntegerOverflow=off
  Cast3 : DataTypeConversion  Commented=on  OutDataTypeStr=single  SaturateOnIntegerOverflow=off  RndMeth=Floor
  Divide : Product  Inputs=*/
  Divide1 : Product  Inputs=*/
  Divide2 : Product  Inputs=**
  LUT_1 : Lookup_n-D  BreakpointsForDimension1=TV.LUT.Yrd_LUT.LUT_vectors.delta_vector  BreakpointsForDimension2=TV.LUT.Yrd_LUT.LUT_vectors.v_vector  Table=single(TV.LUT.Yrd_LUT.LUT_1.ay_matrix)  InternalRulePriority=Speed  RndMeth=Simplest
      settings: InputPortMap=u0,u1
  Saturation : Saturate  UpperLimit=inf  LowerLimit=3
  yrd : Outport
  wires:
  Divide/1 -> Divide2/2
  Saturation/1 -> LUT_1/2, Divide/2  "vx"
  Abs/1 -> LUT_1/1, Divide1/2  "absolute_front_wheel_angle"
  Divide2/1 -> yrd/1  "yrd"
  Divide1/1 -> Divide2/1  "normalized_front_wheel_angle"
  vx/1 -> Saturation/1
  LUT_1/1 -> Divide/1
  front_wheel_angle/1 -> Abs/1, Divide1/1

== system TVModel_Simulation/Subsystem/Subsystem1/Torque Distribution/Reference Tracking/YRD_LUT_2 ==
  front_wheel_angle : Inport
  vx : Inport  Port=2
  Action Port : ActionPort
  Abs : Abs  SaturateOnIntegerOverflow=off
  Cast : DataTypeConversion  Commented=on  OutDataTypeStr=single  SaturateOnIntegerOverflow=off  RndMeth=Floor
  Divide : Product  Inputs=*/
  Divide1 : Product  Inputs=*/
  Divide2 : Product  Inputs=**
  LUT_0 : Lookup_n-D  BreakpointsForDimension1=TV.LUT.Yrd_LUT.LUT_vectors.delta_vector  BreakpointsForDimension2=TV.LUT.Yrd_LUT.LUT_vectors.v_vector  Table=single(TV.LUT.Yrd_LUT.LUT_0.ay_matrix)  InternalRulePriority=Speed  RndMeth=Simplest
      settings: InputPortMap=u0,u1
  Saturation : Saturate  UpperLimit=inf  LowerLimit=3
  yrd : Outport
  wires:
  front_wheel_angle/1 -> Divide1/1, Abs/1
  Saturation/1 -> Divide/2, LUT_0/2  "vx"
  Abs/1 -> Divide1/2, LUT_0/1  "absolute_front_wheel_angle"
  Divide2/1 -> yrd/1  "yrd"
  vx/1 -> Saturation/1
  Divide/1 -> Divide2/2
  Divide1/1 -> Divide2/1  "normalized_front_wheel_angle"
  LUT_0/1 -> Divide/1

== system TVModel_Simulation/Subsystem/Subsystem1/Torque Distribution/Reference Tracking/YRD_LUT_3 ==
  front_wheel_angle : Inport
  vx : Inport  Port=2
  Action Port : ActionPort
  Abs : Abs  SaturateOnIntegerOverflow=off
  Cast3 : DataTypeConversion  Commented=on  OutDataTypeStr=single  SaturateOnIntegerOverflow=off  RndMeth=Floor
  Divide : Product  Inputs=*/
  Divide1 : Product  Inputs=*/
  Divide2 : Product  Inputs=**
  LUT_1 : Lookup_n-D  BreakpointsForDimension1=TV.LUT.Yrd_LUT.LUT_vectors.delta_vector  BreakpointsForDimension2=TV.LUT.Yrd_LUT.LUT_vectors.v_vector  Table=single(TV.LUT.Yrd_LUT.LUT_1.ay_matrix)  InternalRulePriority=Speed  RndMeth=Simplest
      settings: InputPortMap=u0,u1
  Saturation : Saturate  UpperLimit=inf  LowerLimit=3
  yrd : Outport
  wires:
  front_wheel_angle/1 -> Divide1/1, Abs/1
  LUT_1/1 -> Divide/1
  vx/1 -> Saturation/1
  Divide1/1 -> Divide2/1  "normalized_front_wheel_angle"
  Divide2/1 -> yrd/1  "yrd"
  Abs/1 -> Divide1/2, LUT_1/1  "absolute_front_wheel_angle"
  Saturation/1 -> Divide/2, LUT_1/2  "vx"
  Divide/1 -> Divide2/2

== system TVModel_Simulation/Subsystem/Subsystem1/Torque Limits/Torque Limits Positive/Torque_Curve ==
  omega_wheels : Inport
  voltage [ID380] : Inport  Port=2
  torque_map : Inport  Port=3
  2-D Lookup Table : Lookup_n-D  BreakpointsForDimension1=TV.LV.TORQUE.T_lim_pos.breakpoints1  BreakpointsForDimension2=TV.LV.TORQUE.T_lim_pos.breakpoints2  Table=TV.LV.TORQUE.T_lim_pos.table_data  ExtrapMethod=Clip  InternalRulePriority=Speed  OutDataTypeStr=double  RndMeth=Simplest
      settings: InputPortMap=u0,u1
  Constant : Constant  Value=0
  Constant1 : Constant  Value=TV.LV.TORQUE.T_peak_motor
  Constant2 : Constant  Value=TV.LV.TORQUE.T_nominal_motor
  Gain : Gain  Gain=TV.LV.TORQUE.T_nominal_motor/1000
  Gain4 : Gain  Gain=TV.CAR.Tau*60/(2*pi)
  Low-Pass Filter (Discrete or Continuous) : eeGeneralControl/Low-Pass Filter (Discrete or Continuous)  K=1  T=1/4/pi  B=inf  A=-inf  init_option=Inherited from block input  x0=0  Ts=TV.MPC.T/TV.MPC.N
  Multiport Switch : MultiPortSwitch  DataPortOrder=Specify indices  DataPortIndices={TV.LV.TORQUE.T_peak_setting,TV.LV.TORQUE.T_nominal_setting}  DiagnosticForDefault=None  SaturateOnIntegerOverflow=off  InputSameDT=off
  Saturation Dynamic : simulink/Discontinuities/Saturation Dynamic  OutMin=[]  OutMax=[]  OutDataTypeStr=Inherit: Same as second input  OutDataType=fixdt(1, 16)  OutScaling=2^-10  DoSatur=off
  Saturation1 : Saturate  UpperLimit=+inf  LowerLimit=0
  max_torque_available : Outport
  wires:
  Low-Pass Filter (Discrete or Continuous)/1 -> Saturation Dynamic/2
  omega_wheels/1 -> Gain4/1
  Constant/1 -> Saturation Dynamic/3
  torque_map/1 -> Multiport Switch/1
  Constant1/1 -> Multiport Switch/2
  Constant2/1 -> Multiport Switch/3
  Multiport Switch/1 -> Saturation Dynamic/1  "torque map selected"
  Saturation1/1 -> 2-D Lookup Table/1
  voltage [ID380]/1 -> 2-D Lookup Table/2
  Gain/1 -> Low-Pass Filter (Discrete or Continuous)/1
  2-D Lookup Table/1 -> Gain/1
  Gain4/1 -> Saturation1/1  "RPM_Motors"
  Saturation Dynamic/1 -> max_torque_available/1

== system TVModel_Simulation/Subsystem/Subsystem1/Torque Limits/Torque Limits Regen/Torque Curve ==
  omega_wheels : Inport
  voltage [ID380] : Inport  Port=2
  torque_map : Inport  Port=3
  1-D Lookup Table : Lookup_n-D  NumberOfTableDimensions=1  BreakpointsForDimension1=uint16(TV.LUT.Power_LUT.Power.LUT_regen.X)  Table=uint16(abs(TV.LUT.Power_LUT.Power.LUT_regen.Y)*10)  InternalRulePriority=Speed  RndMeth=Simplest
  2-D Lookup Table1 : Lookup_n-D  BreakpointsForDimension1=TV.LV.TORQUE.T_lim_pos.breakpoints1  BreakpointsForDimension2=TV.LV.TORQUE.T_lim_pos.breakpoints2  Table=TV.LV.TORQUE.T_lim_pos.table_data  ExtrapMethod=Clip  InternalRulePriority=Speed  OutDataTypeStr=double  RndMeth=Simplest
      settings: InputPortMap=u0,u1
  Constant : Constant  Value=0
  Constant1 : Constant  Value=TV.LV.TORQUE.T_peak_motor
  Constant2 : Constant  Value=TV.LV.TORQUE.T_nominal_motor
  Gain : Gain  Gain=TV.LV.TORQUE.T_nominal_motor/1000
  Gain4 : Gain  Gain=TV.CAR.Tau*60/(2*pi)
  Min : MinMax  Inputs=2
  Multiport Switch : MultiPortSwitch  DataPortOrder=Specify indices  DataPortIndices={TV.LV.TORQUE.T_peak_setting,TV.LV.TORQUE.T_nominal_setting}  DiagnosticForDefault=None  SaturateOnIntegerOverflow=off  InputSameDT=off
  Rate Limiter : RateLimiter  RisingSlewLimit=2*TV.LV.TORQUE.T_peak_motor  FallingSlewLimit=-inf  SampleTimeMode=inherited  InitialCondition=TV.LV.TORQUE.T_peak_motor
  Saturation Dynamic : simulink/Discontinuities/Saturation Dynamic  OutMin=[]  OutMax=[]  OutDataTypeStr=Inherit: Same as second input  OutDataType=fixdt(1, 16)  OutScaling=2^-10  DoSatur=off
  Saturation1 : Saturate  UpperLimit=+inf  LowerLimit=0
  max_torque_available : Outport
  wires:
  omega_wheels/1 -> Gain4/1
  Saturation Dynamic/1 -> Rate Limiter/1
  Gain/1 -> Saturation Dynamic/2
  Constant2/1 -> Multiport Switch/3
  Multiport Switch/1 -> Saturation Dynamic/1  "torque map selected"
  Constant/1 -> Saturation Dynamic/3
  2-D Lookup Table1/1 -> Min/2
  Saturation1/1 -> 2-D Lookup Table1/1, 1-D Lookup Table/1
  voltage [ID380]/1 -> 2-D Lookup Table1/2
  torque_map/1 -> Multiport Switch/1
  Constant1/1 -> Multiport Switch/2
  1-D Lookup Table/1 -> Min/1
  Min/1 -> Gain/1
  Gain4/1 -> Saturation1/1  "RPM_Motors"
  Rate Limiter/1 -> max_torque_available/1  "max_torque_available"

== system TVModel_Simulation/Subsystem/Subsystem1/Torque Limits/Torque Request/T_Req_Acceleration ==
  throttle : Inport
  torque_map : Inport  Port=2
  Constant : Constant  Value=0
  Constant1 : Constant
  Constant2 : Constant  Value=0
  Data Store General_Params : DataStoreRead  DataStoreName=General_Params  DataStoreElements=General_Params.ThrottleThresh  IndexOptions=Index vector (dialog)  Indices=1  OutputSizes=1
  Data Store General_Params1 : DataStoreRead  DataStoreName=General_Params  DataStoreElements=General_Params.ThrottleThresh  IndexOptions=Index vector (dialog)  Indices=1  OutputSizes=1
  Less Than : RelationalOperator  Operator=>  OutDataTypeStr=boolean  RndMeth=Simplest  InputSameDT=off
  Map_Selector : MultiPortSwitch  DataPortOrder=Specify indices  DataPortIndices={TV.LV.TORQUE.T_peak_setting,TV.LV.TORQUE.T_nominal_setting}  DiagnosticForDefault=None  SaturateOnIntegerOverflow=off  InputSameDT=off
  Mux : Mux  Inputs=3
  Switch : Switch  Criteria=u2 > Threshold  SaturateOnIntegerOverflow=off  InputSameDT=off
  T_nominal_wheel_LUT : Lookup_n-D  NumberOfTableDimensions=1  BreakpointsForDimension1Source=Input port  BreakpointsForDimension1=[-5:5]  Table=[0,0, 4*TV.LV.TORQUE.T_nominal_wheel]  InternalRulePriority=Speed  RndMeth=Simplest
      settings: InputPortMap=u0,p5
  T_peak_wheel_LUT : Lookup_n-D  NumberOfTableDimensions=1  BreakpointsForDimension1Source=Input port  BreakpointsForDimension1=[-5:5]  Table=[0,0, 4*TV.LV.TORQUE.T_peak_wheel]  InternalRulePriority=Speed  RndMeth=Simplest
      settings: InputPortMap=u0,p5
  "t_req " : Outport
  wires:
  throttle/1 -> T_nominal_wheel_LUT/1, Less Than/1, T_peak_wheel_LUT/1  "throttle"
  Map_Selector/1 -> Switch/1  "t"
  Data Store General_Params1/1 -> Less Than/2  "throttle_thresh"
  Less Than/1 -> Switch/2  "throttle"
  Switch/1 -> "t_req "/1
  Constant/1 -> Switch/3
  T_nominal_wheel_LUT/1 -> Map_Selector/3
  T_peak_wheel_LUT/1 -> Map_Selector/2
  torque_map/1 -> Map_Selector/1  "torque_map"
  Mux/1 -> T_nominal_wheel_LUT/2, T_peak_wheel_LUT/2
  Data Store General_Params/1 -> Mux/2  "throttle_thresh"
  Constant1/1 -> Mux/3
  Constant2/1 -> Mux/1

== system TVModel_Simulation/Subsystem/Subsystem1/Torque Limits/Torque Request/T_Req_Braking ==
  brake : Inport
  1-D Lookup Table : Lookup_n-D  NumberOfTableDimensions=1  BreakpointsForDimension1Source=Input port  BreakpointsForDimension1=[-5:5]  Table=[0,1]  InternalRulePriority=Speed  RndMeth=Simplest
      settings: InputPortMap=u0,p5
  Constant : Constant
  Data Store Read : DataStoreRead  DataStoreName=General_Params  DataStoreElements=General_Params.BrakeThresh  IndexOptions=Index vector (dialog)  Indices=1  OutputSizes=1
  Gain_Max_Torque_Needed : Gain  Gain=-4*TV.LV.TORQUE.T_nominal_wheel
  Mux : Mux  Inputs=2
  Saturation_Brake : Saturate  UpperLimit=1  LowerLimit=0
  "t_req " : Outport
  wires:
  Gain_Max_Torque_Needed/1 -> "t_req "/1  "t_req"
  brake/1 -> 1-D Lookup Table/1  "brake"
  1-D Lookup Table/1 -> Saturation_Brake/1  "brake"
  Saturation_Brake/1 -> Gain_Max_Torque_Needed/1  "brake"
  Data Store Read/1 -> Mux/1
  Constant/1 -> Mux/2
  Mux/1 -> 1-D Lookup Table/2

== system TVModel_Simulation/Subsystem/Subsystem1/Torque Distribution/MPC/     Output vector reference/Bus y_ref ==
  u : Inport
  C Function : CFunction  OutputCode=|
      | int i,j;
      | for (i = 0; i < N; i++) {
      |  for (j = 0; j < ny; j++) {
      |   out_x[i*ny+j] = in_x[j];
      |  }
      | }
  Constant1 : Constant  Value=TV.MPC.N  OutDataTypeStr=uint8  SampleTime=TV.MPC.T/TV.MPC.N
  Constant3 : Constant  Value=TV.MPC.ny  OutDataTypeStr=uint8  SampleTime=TV.MPC.T/TV.MPC.N
  Rate Transition3 : RateTransition  OutPortSampleTime=TV.MPC.T/TV.MPC.N
  y : Outport
  wires:
  u/1 -> Rate Transition3/1
  Constant1/1 -> C Function/2
  Constant3/1 -> C Function/3
  Rate Transition3/1 -> C Function/1
  C Function/1 -> y/1

== system TVModel_Simulation/Subsystem/Subsystem1/Torque Distribution/MPC/ Parameter Bus /Bus p ==
  In : Inport
  C Function : CFunction  OutputCode=|
      | int i,j;
      | for (i = 0; i < N; i++) {
      |  for (j = 0; j < np; j++) {
      |   out_x[i*np+j] = in_x[j];
      |  }
      | }
  Constant1 : Constant  Value=TV.MPC.N + 1  OutDataTypeStr=uint8  SampleTime=TV.MPC.T/TV.MPC.N
  Constant3 : Constant  Value=TV.MPC.np  OutDataTypeStr=uint8  SampleTime=TV.MPC.T/TV.MPC.N
  Rate Transition3 : RateTransition  OutPortSampleTime=TV.MPC.T/TV.MPC.N
  Out : Outport
  wires:
  Constant1/1 -> C Function/2
  C Function/1 -> Out/1
  Constant3/1 -> C Function/3
  Rate Transition3/1 -> C Function/1
  In/1 -> Rate Transition3/1

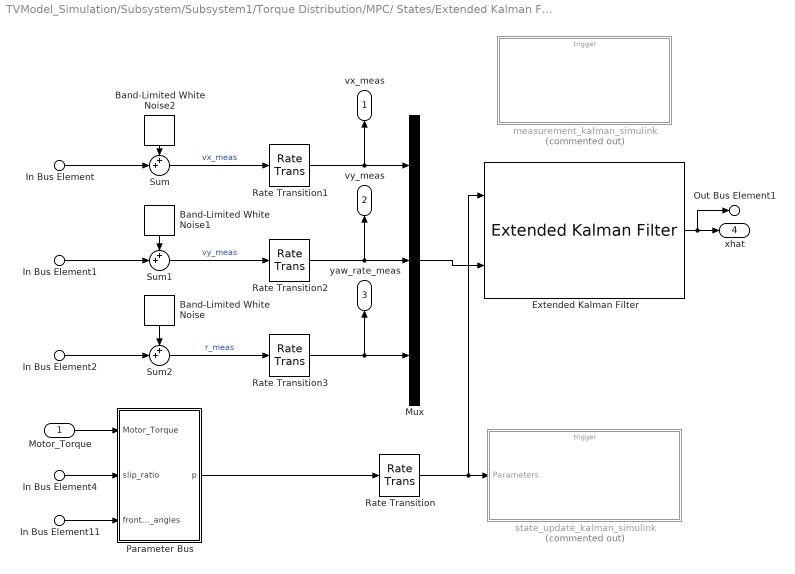
== system TVModel_Simulation/Subsystem/Subsystem1/Torque Distribution/MPC/ States/Extended Kalman Filter ==
  Motor_Torque : Inport
  In Bus Element4 : Inport  Port=2  PortName=slip_ratio
  In Bus Element : Inport  Port=3  PortName=dynamics_data  Element=vx
  In Bus Element1 : Inport  Port=3  PortName=dynamics_data  Element=vy
  In Bus Element2 : Inport  Port=3  PortName=dynamics_data  Element=yaw_rate
  In Bus Element11 : Inport  Port=4  PortName=front_wheel_angles
  " Parameter Bus " : Subsystem
  Band-Limited White Noise : simulink/Sources/Band-Limited White Noise  Cov=0.00005  Ts=0.01  seed=[23341]
  Band-Limited White Noise1 : simulink/Sources/Band-Limited White Noise  Cov=0.000001  Ts=0.01  seed=[23341]
  Band-Limited White Noise2 : simulink/Sources/Band-Limited White Noise  Cov=0.00001  Ts=0.01  seed=[85]
  Extended Kalman Filter : sharedTrackingLibrary/Extended Kalman Filter  StateTransitionFcn=state_update_kalman  HasStateTransitionJacobianFcn=off  HasAdditiveProcessNoise=Additive  ProcessNoise=diag(0.1*[0.1,0.1,0.1])  HasTimeVaryingProcessNoise=off  HasStateTransitionFcnExtraArgument=1  InitialState=[0,0,0];  InitialStateCovariance=diag(0.1*[0.1,0.1,0.1])  MeasurementFcn1=measurement_kalman  HasMeasurementJacobianFcn1=off  HasMeasurementEnablePort1=off  HasAdditiveMeasurementNoise1=Additive  MeasurementNoise1=diag(0.1*[0.01,0.01,1])  HasTimeVaryingMeasurementNoise1=off  HasMeasurementFcnExtraArgument1=0  HasMeasurementWrapping1=off  MeasurementFcn2=myMeasurementFcn  HasMeasurementJacobianFcn2=off  HasMeasurementEnablePort2=off  HasAdditiveMeasurementNoise2=Additive  MeasurementNoise2=1  HasTimeVaryingMeasurementNoise2=off  HasMeasurementFcnExtraArgument2=0  HasMeasurementWrapping2=off  MeasurementFcn3=myMeasurementFcn  HasMeasurementJacobianFcn3=off  HasMeasurementEnablePort3=off  HasAdditiveMeasurementNoise3=Additive  MeasurementNoise3=1  HasTimeVaryingMeasurementNoise3=off  HasMeasurementFcnExtraArgument3=0  HasMeasurementWrapping3=off  MeasurementFcn4=myMeasurementFcn  HasMeasurementJacobianFcn4=off  HasMeasurementEnablePort4=off  HasAdditiveMeasurementNoise4=Additive  MeasurementNoise4=1  HasTimeVaryingMeasurementNoise4=off  HasMeasurementFcnExtraArgument4=0  HasMeasurementWrapping4=off  MeasurementFcn5=myMeasurementFcn  HasMeasurementJacobianFcn5=off  HasMeasurementEnablePort5=off  HasAdditiveMeasurementNoise5=Additive  MeasurementNoise5=1  HasTimeVaryingMeasurementNoise5=off  HasMeasurementFcnExtraArgument5=0  HasMeasurementWrapping5=off  EnableMultirate=off  StateTransitionFcnSampleTime=1  MeasurementFcn1SampleTime=1  MeasurementFcn2SampleTime=1  MeasurementFcn3SampleTime=1  MeasurementFcn4SampleTime=1  MeasurementFcn5SampleTime=1  UseCurrentEstimator=on  OutputStateCovariance=off  DataType=double  SampleTime=TV.MPC.T/TV.MPC.N  NumberOfMeasurements=1
      settings: SourceProductBaseCode=TF,AE,PW,CT,DR,ID,LP,NV,AR,RO,RR,UV,VE
  Mux : Mux  Inputs=3
  Rate Transition{,1..3} (4 alike) : RateTransition  OutPortSampleTime=TV.MPC.T/TV.MPC.N
  Sum : Sum  Inputs=++|
  Sum1 : Sum  Inputs=++|
  Sum2 : Sum  Inputs=++|
  measurement_kalman_simulink : Subsystem  Commented=on  TreatAsAtomicUnit=on
  state_update_kalman_simulink : Subsystem  Commented=on  TreatAsAtomicUnit=on
  vx_meas : Outport
  vy_meas : Outport  Port=2
  yaw_rate_meas : Outport  Port=3
  xhat : Outport  Port=4
  Out Bus Element1 : Outport  Port=5  PortName=TV_Info  Element=xhat_ext
  wires:
  In Bus Element11/1 -> " Parameter Bus "/3(front_wheel_angles)
  Motor_Torque/1 -> " Parameter Bus "/1(Motor_Torque)
  In Bus Element4/1 -> " Parameter Bus "/2(slip_ratio)
  Rate Transition3/1 -> yaw_rate_meas/1, Mux/3
  Sum2/1 -> Rate Transition3/1  "r_meas"
  Rate Transition2/1 -> vy_meas/1, Mux/2
  Sum1/1 -> Rate Transition2/1  "vy_meas"
  Sum/1 -> Rate Transition1/1  "vx_meas"
  Rate Transition1/1 -> Mux/1, vx_meas/1
  Band-Limited White Noise/1 -> Sum2/1
  In Bus Element2/1 -> Sum2/2
  Band-Limited White Noise1/1 -> Sum1/1
  In Bus Element1/1 -> Sum1/2
  Band-Limited White Noise2/1 -> Sum/1
  In Bus Element/1 -> Sum/2
  Extended Kalman Filter/1 -> Out Bus Element1/1, xhat/1
  Mux/1 -> Extended Kalman Filter/2
  " Parameter Bus "/1(p) -> Rate Transition/1
  Rate Transition/1 -> Extended Kalman Filter/1, state_update_kalman_simulink/1(Parameters)

== system TVModel_Simulation/Subsystem/Subsystem1/Torque Distribution/MPC/ States/Yrd 0 When Steering 0 ==
  yaw_rate_desired_LUT : Inport
  front_steer_angle : Inport  Port=2
  vx : Inport  Port=3
  Abs : Abs  SaturateOnIntegerOverflow=off
  Constant5 : Constant  Value=0
  Linear Activation : MATLAB Function  TreatAsAtomicUnit=on
  Steer Limit : Subsystem
      mask Display: image('Mask_Icon\steering-wheel.png'); % Use "Edit Image" on toolstrip to change.
  yaw_rate_desired : Outport
  wires:
  Constant5/1 -> Linear Activation/3(in_2)
  yaw_rate_desired_LUT/1 -> Linear Activation/1(in_1)
  Linear Activation/1(out) -> yaw_rate_desired/1
  Steer Limit/1(steer_limit) -> Linear Activation/2(epsilon)
  front_steer_angle/1 -> Abs/1
  vx/1 -> Steer Limit/2(Inport)
  Abs/1 -> Steer Limit/1(front_wheel_angle)

== system TVModel_Simulation/Subsystem/Subsystem1/Torque Distribution/MPC/Faults detection/Power flag ==
  Motor_Torque : Inport
  dynamics_data : Inport  Port=2
  Constant : Constant  Value=79000
  Constant1 : Constant  Value=0
  Constant2 : Constant  Value=-34000
  Efficiency limit : Subsystem
  Less Than : RelationalOperator  OutDataTypeStr=boolean  RndMeth=Simplest  InputSameDT=off
  Less Than1 : RelationalOperator  OutDataTypeStr=boolean  RndMeth=Simplest  InputSameDT=off
  Less Than2 : RelationalOperator  Operator=<=  OutDataTypeStr=boolean  RndMeth=Simplest  InputSameDT=off
  Sum1 : Sum  Inputs=+
  Switch : Switch  Criteria=u2 > Threshold  SaturateOnIntegerOverflow=off  InputSameDT=off
  Output : Outport
  wires:
  Switch/1 -> Output/1
  Constant2/1 -> Less Than2/2
  Less Than2/1 -> Switch/3
  Less Than/1 -> Switch/1
  Less Than1/1 -> Switch/2
  Constant1/1 -> Less Than1/2
  Motor_Torque/1 -> Efficiency limit/1(Motor_Torque)
  dynamics_data/1 -> Efficiency limit/2(dynamics_data)
  Efficiency limit/1(Limit) -> Sum1/1  "Limit"
  Constant/1 -> Less Than/2
  Sum1/1 -> Less Than1/1, Less Than/1, Less Than2/1  "Power"

== system TVModel_Simulation/Subsystem/Subsystem1/Torque Distribution/MPC/Faults detection/Subsystem ==
  T : Inport
  In2 : Inport  Port=2
  In3 : Inport  Port=3
  Constant : Constant  Value=-35000
  Constant1 : Constant  Value=TV.LV.efficiency_LUT.Eta
  Constant2 : Constant  Value=TV.LV.efficiency_LUT.Omega
  Constant3 : Constant  Value=TV.LV.efficiency_LUT.Torque
  Constant4 : Constant  Value=TV.LV.GENERAL.BrakeThresh
  Constant5 : Constant  Value=80000
  Gain1 : Gain  Gain=TV.CAR.Tau
  Less Than1 : RelationalOperator  Operator=<  OutDataTypeStr=boolean  RndMeth=Simplest  InputSameDT=off
  MATLAB Function : MATLAB Function  TreatAsAtomicUnit=on
  Switch1 : Switch  Criteria=u2 > Threshold  SaturateOnIntegerOverflow=off  InputSameDT=off
  Terminator1 : Terminator
  Terminator2 : Terminator
  Output : Outport
  wires:
  In3/1 -> Less Than1/2
  T/1 -> MATLAB Function/1(T)
  In2/1 -> Gain1/1
  Switch1/1 -> MATLAB Function/2(Plim)
  Less Than1/1 -> Switch1/2, MATLAB Function/7(brake_flag)
  Constant4/1 -> Less Than1/1
  MATLAB Function/1(Tnew) -> Output/1  "Tnew"
  MATLAB Function/2(k) -> Terminator1/1  "k"
  MATLAB Function/3(fx) -> Terminator2/1  "fx"
  Constant2/1 -> MATLAB Function/4(Omega)
  Constant3/1 -> MATLAB Function/5(Torque)
  Constant5/1 -> Switch1/3
  Constant/1 -> Switch1/1
  Constant1/1 -> MATLAB Function/3(Eta)
  Gain1/1 -> MATLAB Function/6(Omega_motors)
